simulink model "position_control_PD_with_Due"  (R2022a)
settings: Solver=FixedStepAuto  StartTime=0.0  StopTime=10  FixedStep=0.01  RelTol=1e-3  EnableMultiTasking=on
undefined symbols (not defined in the file or in its folder): a, b, kd2, kd4, kp2, kp4
libraries: arduinolib x4, arduinosensorlib x1
settings Model: ExtModeTrigDuration=2  Creator=DCLab  LastModifiedBy=LabPC
settings OptimizationCC: EnhancedBackFolding=on  PassReuseOutputArgsAs=Individual arguments  ZeroExternalMemoryAtStartup=off  ZeroInternalMemoryAtStartup=off  MaxStackSize=64  OptimizeBlockOrder=speed  DifferentSizesBufferReuse=on  OptimizationCustomize=off  EfficientTunableParamExpr=on
settings DebuggingCC: ParameterTunabilityLossMsg=error  UnconnectedInputMsg=warning  UnconnectedOutputMsg=warning  UnconnectedLineMsg=warning
settings HardwareCC: ProdBitPerPointer=32  ProdBitPerSizeT=32  ProdBitPerPtrDiffT=32  ProdLargestAtomicInteger=Long  ProdLargestAtomicFloat=Double  ProdWordSize=32  ProdHWDeviceType=ARM Compatible->ARM Cortex
settings SFSimCC: MATLABDynamicMemAlloc=off  SimTargetLang=C++
settings RTWCC: SystemTargetFile=ert.tlc  HardwareBoard=Arduino Due  TemplateMakefile=ert_default_tmf  Toolchain=Arduino ARM  BuildConfiguration=Faster Runs  DLArmComputeVersion=19.05
settings CodeAppCC: ForceParamTrailComments=on  IgnoreCustomStorageClasses=off  OperatorAnnotations=on  SimulinkDataObjDesc=on  SFDataObjDesc=on  InsertBlockDesc=on
settings ERTTargetCC: SupportContinuousTime=on  SupportVariableSizeSignals=on  ExtModeTransport=3  ExtModeStaticAlloc=on  ExtModeStaticAllocSize=24576  ExtModeMexFile=ext_xcp  ExtModeIntrfLevel=Level2 - Open

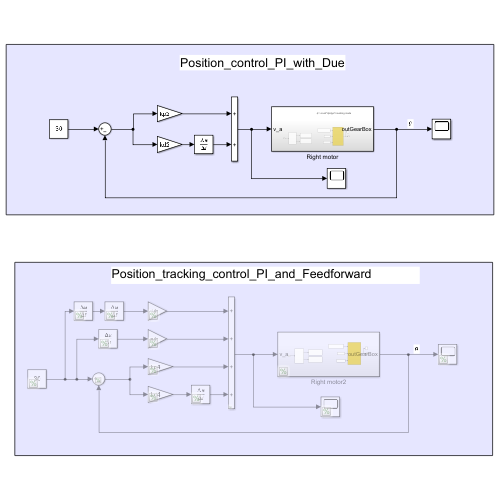
[thumbnail: Simulink's stored preview of the top-level diagram]
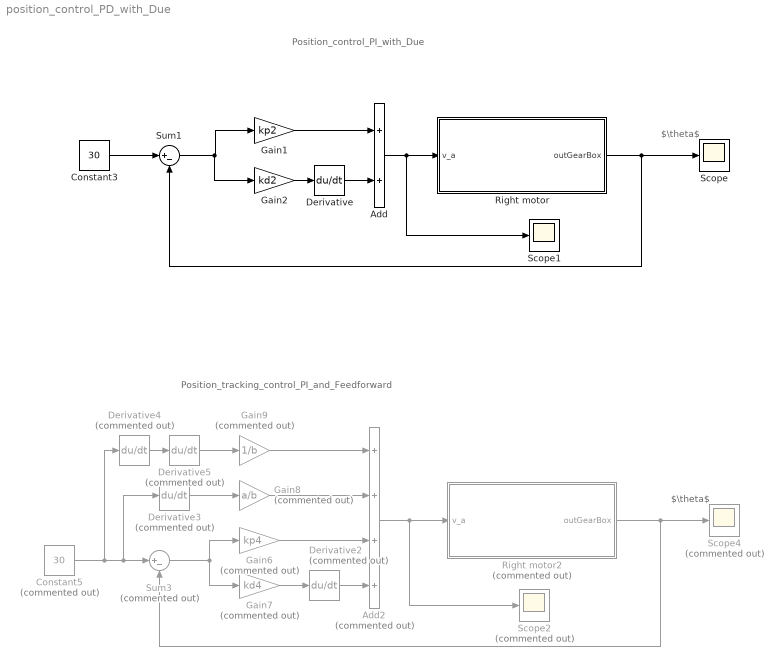
== system position_control_PD_with_Due ==
  note: Position_control_PI_with_Due
  note: $\theta$
  note: $\theta$
  note: Position_tracking_control_PI_and_Feedforward
  Add : Sum
  Add2 : Sum  Commented=on  Inputs=++++
  Constant3 : Constant  Value=30
  Constant5 : Constant  Commented=on  Value=30
  Derivative : Derivative
  Derivative{2..5} (4 alike) : Derivative  Commented=on
  Gain1 : Gain  Gain=kp2
  Gain2 : Gain  Gain=kd2
  Gain6 : Gain  Commented=on  Gain=kp4
  Gain7 : Gain  Commented=on  Gain=kd4
  Gain8 : Gain  Commented=on  Gain=a/b
  Gain9 : Gain  Commented=on  Gain=1/b
  Right motor : Subsystem
  Right motor2 : Subsystem  Commented=on
  Scope : Scope
  Scope1 : Scope
  Scope2 : Scope  Commented=on
  Scope4 : Scope  Commented=on
  Sum1 : Sum  Inputs=|+-
  Sum3 : Sum  Commented=on  Inputs=|+-
  wires:
  Gain2/1 -> Derivative/1
  Sum1/1 -> Gain2/1, Gain1/1
  Derivative/1 -> Add/2
  Gain1/1 -> Add/1
  Add/1 -> Scope1/1, Right motor/1(v_a)
  Right motor/1(outGearBox) -> Sum1/2, Scope/1
  Constant3/1 -> Sum1/1
  Sum3/1 -> Gain6/1, Gain7/1
  Gain9/1 -> Add2/1
  Derivative2/1 -> Add2/4
  Gain6/1 -> Add2/3
  Constant5/1 -> Derivative4/1, Derivative3/1, Sum3/1
  Gain7/1 -> Derivative2/1
  Gain8/1 -> Add2/2
  Derivative3/1 -> Gain8/1
  Derivative4/1 -> Derivative5/1
  Derivative5/1 -> Gain9/1
  Right motor2/1(outGearBox) -> Sum3/2, Scope4/1
  Add2/1 -> Scope2/1, Right motor2/1(v_a)

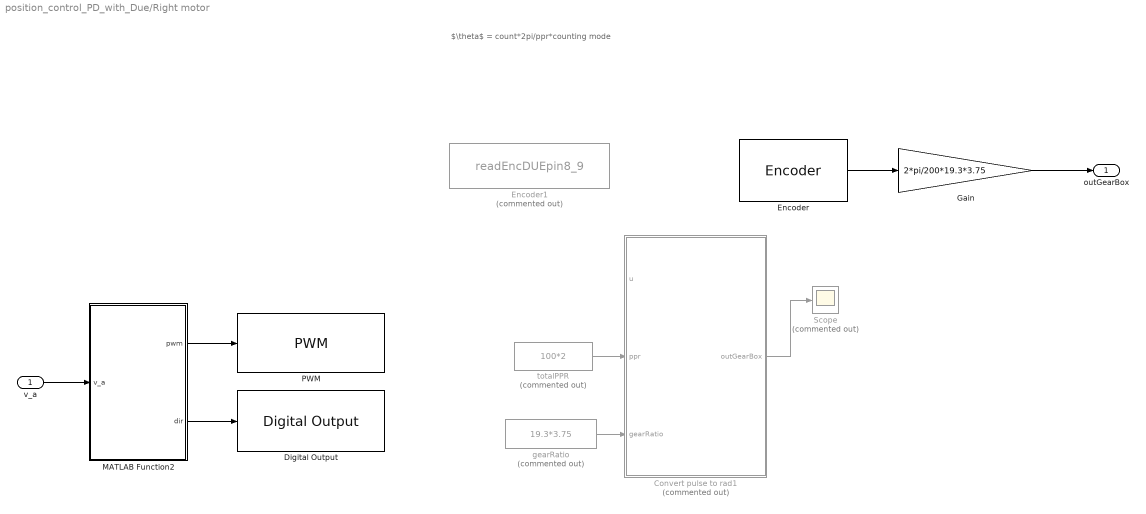
== system position_control_PD_with_Due/Right motor ==
  note: $\theta$ = count*2pi/ppr*counting mode
  v_a : Inport
  Convert pulse to rad1 : MATLAB Function  Commented=on  TreatAsAtomicUnit=on
  Digital Output : arduinolib/Digital Output  pinNumber=7  Direction=output  blockPlatform=arduino
  Encoder : arduinosensorlib/Encoder  InputA=2  InputB=3  Mode=No reset  SampleTime=-1
      settings: SourceProductBaseCode=ARDUINO
  Encoder1 : S-Function  Commented=on  InitFcn=try, set_param(gcb,'FunctionName','readEncDUEpin8_9'), end  FunctionName=readEncDUEpin8_9  SFunctionModules=readEncDUEpin8_9_wrapper  SFunctionDeploymentMode=off  EnableBusSupport=off  mask(S-Function Builder){}
      mask help: Simulink:masks:SFunctionBuilder_MD
      mask init:
      | val = [[.9  0.75 0.75 1 1 .9 .9 1]',[1 1 0.75 0.75 .9 .9 1 .9]'];try , sys = get_param(gcb,'SfunBuilderFcnName');if isempty(sys), sys = get_param(gcb,'FunctionName'); end,catch, sys = get_param(gcb,'FunctionName'); end
      settings: CopyFcn=set_param(gcbh,'LinkStatus','none')  PreSaveFcn=try, set_param(gcb,'FunctionName','readEncDUEpin8_9'), end  OpenFcn=sfunctionwizard(gcbh)
      mask Display:
      | plot(val(:,1),val(:,2))
      | disp(sys)
      | port_label('output',1,'count')
  Gain : Gain  Gain=2*pi/200*19.3*3.75
  MATLAB Function2 : MATLAB Function  TreatAsAtomicUnit=on
  PWM : arduinolib/PWM  pinNumber=6  frequencyType=Default  desiredFrequency=490.2  achievableFrequency=490.2
  Scope : Scope  Commented=on
  gearRatio : Constant  Commented=on  Value=19.3*3.75
  totalPPR : Constant  Commented=on  Value=100*2
  outGearBox : Outport
  wires:
  totalPPR/1 -> Convert pulse to rad1/2(ppr)
  v_a/1 -> MATLAB Function2/1(v_a)
  MATLAB Function2/2(dir) -> Digital Output/1
  MATLAB Function2/1(pwm) -> PWM/1
  gearRatio/1 -> Convert pulse to rad1/3(gearRatio)
  Convert pulse to rad1/1(outGearBox) -> Scope/1
  Encoder/1 -> Gain/1
  Gain/1 -> outGearBox/1

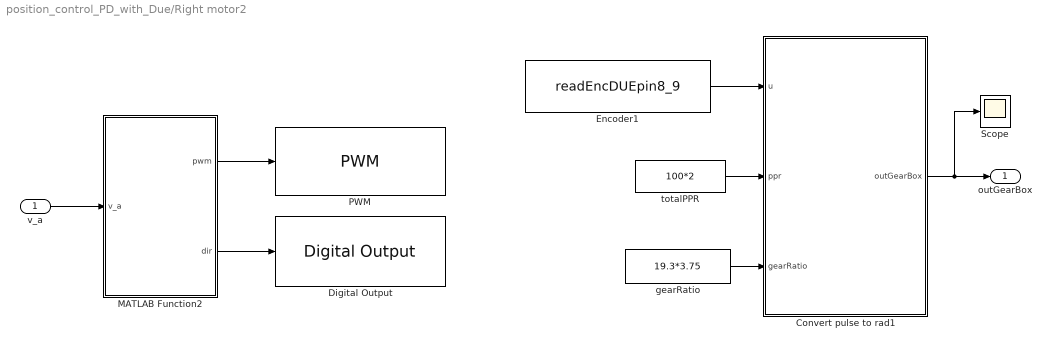
== system position_control_PD_with_Due/Right motor2 ==
  v_a : Inport
  Convert pulse to rad1 : MATLAB Function  TreatAsAtomicUnit=on
  Digital Output : arduinolib/Digital Output  pinNumber=7  Direction=output  blockPlatform=arduino
  Encoder1 : S-Function  InitFcn=try, set_param(gcb,'FunctionName','readEncDUEpin8_9'), end  FunctionName=readEncDUEpin8_9  SFunctionModules=readEncDUEpin8_9_wrapper  SFunctionDeploymentMode=off  EnableBusSupport=off  mask(S-Function Builder){}
      mask help: Simulink:masks:SFunctionBuilder_MD
      mask init: same as position_control_PD_with_Due/Right motor/Encoder1
      settings: CopyFcn=set_param(gcbh,'LinkStatus','none')  PreSaveFcn=try, set_param(gcb,'FunctionName','readEncDUEpin8_9'), end  OpenFcn=sfunctionwizard(gcbh)
      mask Display:
      | plot(val(:,1),val(:,2))
      | disp(sys)
      | port_label('output',1,'count')
  MATLAB Function2 : MATLAB Function  TreatAsAtomicUnit=on
  PWM : arduinolib/PWM  pinNumber=6  frequencyType=Default  desiredFrequency=490.2  achievableFrequency=490.2
  Scope : Scope
  gearRatio : Constant  Value=19.3*3.75
  totalPPR : Constant  Value=100*2
  outGearBox : Outport
  wires:
  totalPPR/1 -> Convert pulse to rad1/2(ppr)
  v_a/1 -> MATLAB Function2/1(v_a)
  MATLAB Function2/2(dir) -> Digital Output/1
  MATLAB Function2/1(pwm) -> PWM/1
  gearRatio/1 -> Convert pulse to rad1/3(gearRatio)
  Convert pulse to rad1/1(outGearBox) -> Scope/1, outGearBox/1
  Encoder1/1 -> Convert pulse to rad1/1(u)

== matlab function position_control_PD_with_Due/Right motor2/Convert pulse to rad1 ==
  settings: updateMethod=DISCRETE
  data: u input; ppr input; gearRatio input; outGearBox output
function outGearBox = fcn(u,ppr,gearRatio)

persistent counter_num over_flag
if(isempty(counter_num)), counter_num = 0;end
if(isempty(over_flag)), over_flag = 0;end
pulse2radian = 2*pi/ppr; % 1 pulse = ?? radian

if(double(u) - counter_num > 40000), over_flag = over_flag-1;
elseif(double(u) - counter_num < -40000), over_flag = over_flag+1;
end

inGearBox = (double(u)+over_flag*(2^32 -1))*pulse2radian; 
outGearBox = inGearBox/gearRatio;
counter_num = double(u) ;

== matlab function position_control_PD_with_Due/Right motor2/MATLAB Function2 ==
  data: v_a input; pwm output; dir output
function [pwm,dir] = fcn(v_a)

vmax = 22.9;
%vmax = 10;
pwm_cal = v_a*254/vmax;
if pwm_cal > 0
    pwm = pwm_cal;
    dir = 0;
elseif pwm_cal < 0
    pwm = abs(pwm_cal);
    dir = 1;
else
    pwm = 0;
    dir = 0;
end

== matlab function position_control_PD_with_Due/Right motor/MATLAB Function2 ==
  data: v_a input; pwm output; dir output
function [pwm,dir] = fcn(v_a)

vmax = 22.9;
pwm_cal = v_a*254/vmax;
if pwm_cal > 0
    pwm = pwm_cal;
    dir = 0;
elseif pwm_cal < 0
    pwm = abs(pwm_cal);
    dir = 1;
else
    pwm = 0;
    dir = 0;
end

== matlab function position_control_PD_with_Due/Right motor/Convert pulse to rad1 ==
  settings: updateMethod=DISCRETE
  data: u input; ppr input; gearRatio input; outGearBox output
function outGearBox = fcn(u,ppr,gearRatio)

persistent counter_num over_flag
if(isempty(counter_num)), counter_num = 0;end
if(isempty(over_flag)), over_flag = 0;end
pulse2radian = 2*pi/ppr; % 1 pulse = ?? radian

if(double(u) - counter_num > 40000), over_flag = over_flag-1;
elseif(double(u) - counter_num < -40000), over_flag = over_flag+1;
end

inGearBox = (double(u)+over_flag*(2^32 -1))*pulse2radian; 
outGearBox = inGearBox/gearRatio;
counter_num = double(u) ;
